simulink model "funkcia23"  (R2020a)
settings: Solver=VariableStepAuto  StartTime=0.0  StopTime=10.0  RelTol=1e-3
libraries: simulink x1
settings Model: Creator=xacha  LastModifiedBy=xacha

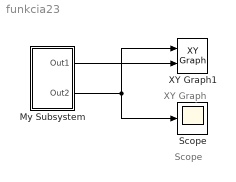
== system funkcia23 ==
  note: Scope
  note: XY Graph
  My Subsystem : Subsystem  mask{a=0, c=1, constant3=3}
      mask prompts: a "input a"; c "input c=1"; constant3 "input constant=3"
      mask DialogControl DescGroupVar Prompt: Subsystem For All Values
      mask DialogControl DescTextVar Prompt: y"-(3*c*y')-(a*c*y)=x*sin(x)
      mask DialogControl ParameterGroupVar Prompt: Input Your Values
  Scope : Scope
  XY Graph1 : simulink/Sinks/XY Graph  xmin=-0.5  xmax=0.8  ymin=-2  ymax=2  st=-1
  wires:
  My Subsystem/1(Out1) -> XY Graph1/2
  My Subsystem/2(Out2) -> Scope/1, XY Graph1/1

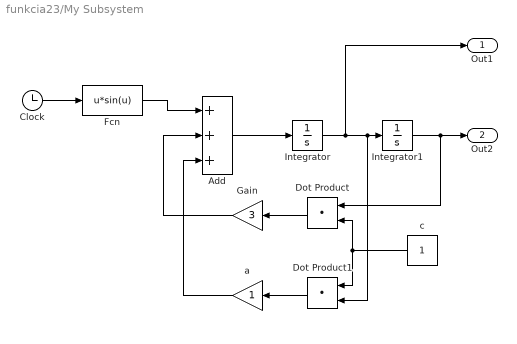
== system funkcia23/My Subsystem ==
  Add : Sum  Inputs=+++
  Clock : Clock
  Dot Product : DotProduct  InputSameDT=on  OutDataTypeStr=Inherit: Inherit via internal rule
  Dot Product1 : DotProduct  InputSameDT=on  OutDataTypeStr=Inherit: Inherit via internal rule
  Fcn : Fcn  Expr=u*sin(u)
  Gain : Gain  Gain=3  mask{constant3=0}
      mask prompts: constant3 "constant 3"
  Integrator : Integrator
  Integrator1 : Integrator
  a : Gain  mask{a=0}
      mask prompts: a "input a"
  c : Constant  mask{c=0}
      mask prompts: c "input c"
  Out1 : Outport  VectorParamsAs1DForOutWhenUnconnected=off
  Out2 : Outport  Port=2  VectorParamsAs1DForOutWhenUnconnected=off
  wires:
  Dot Product/1 -> Gain/1
  Gain/1 -> Add/2
  a/1 -> Add/3
  Dot Product1/1 -> a/1
  c/1 -> Dot Product1/1, Dot Product/2
  Integrator1/1 -> Out2/1, Dot Product/1
  Integrator/1 -> Out1/1, Integrator1/1, Dot Product1/2
  Fcn/1 -> Add/1
  Add/1 -> Integrator/1
  Clock/1 -> Fcn/1
